simulink model "SimulNro1_20230617"  (R2022b)
settings: Solver=ode4  StartTime=0.0  StopTime=1  FixedStep=.001  RelTol=1e-3
values from neighbouring files (symbols this model uses):
  A1 = [-1 0;0 -1]    [StateSpace20240624.m]
  B1 = [1;1]    [StateSpace20240624.m]
  K1 = db2mag(41.6)*zpk(inv(Pmp)/s)    [Problema6.m]    (also in StateSpace20240624.m = acker(A1,B1,[-10 -10]))
libraries: cstblocks x2
settings Model: Creator=aghersin  LastModifiedBy=aghersin

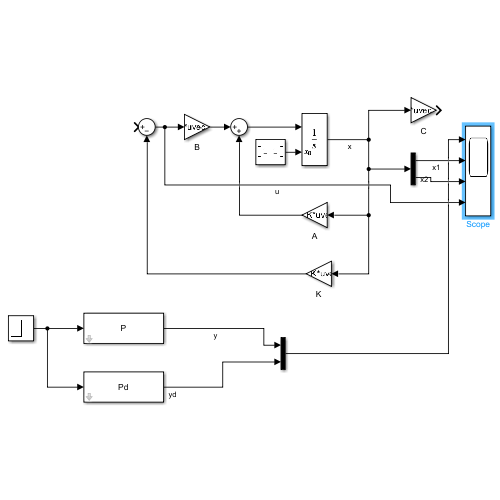
[thumbnail: Simulink's stored preview of the top-level diagram]
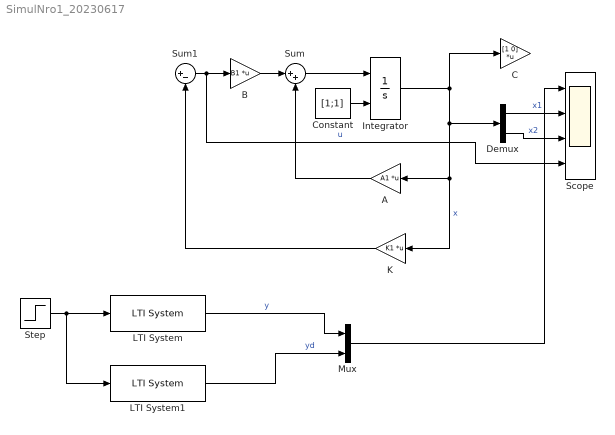
== system SimulNro1_20230617 ==
  A : Gain  Gain=A1  Multiplication=Matrix(K*u) (u vector)
  B : Gain  Gain=B1  Multiplication=Matrix(K*u) (u vector)
  C : Gain  Gain=[1 0]  Multiplication=Matrix(K*u) (u vector)
  Constant : Constant  Value=[1;1]
  Demux : Demux  Outputs=2
  Integrator : Integrator  InitialConditionSource=external
  K : Gain  Gain=K1  Multiplication=Matrix(K*u) (u vector)
  LTI System : cstblocks/LTI System  sys=P  IC=[]
  LTI System1 : cstblocks/LTI System  sys=Pd  IC=[]
  Mux : Mux  Inputs=2
  Scope : Scope  NumInputPorts=4
  Step : Step  Time=.1  SampleTime=0
  Sum : Sum  Inputs=|++
  Sum1 : Sum  Inputs=|+-
  wires:
  Integrator/1 -> C/1, A/1, K/1, Demux/1  "x"
  A/1 -> Sum/2
  B/1 -> Sum/1
  Sum/1 -> Integrator/1
  Constant/1 -> Integrator/2
  Sum1/1 -> Scope/4, B/1  "u"
  K/1 -> Sum1/2
  Demux/1 -> Scope/2  "x1"
  Demux/2 -> Scope/3  "x2"
  Step/1 -> LTI System1/1, LTI System/1
  LTI System/1 -> Mux/1  "y"
  LTI System1/1 -> Mux/2  "yd"
  Mux/1 -> Scope/1
